simulink model "magnetometer"  (R2020b)
settings: Solver=VariableStepAuto  StartTime=0.0  StopTime=10.0  RelTol=1e-3
model mask{m_sf_cc=[1, 0, 0; 0, 1, 0; 0, 0, 1], m_bias=[0 0 0], m_noise=[0 0 0], m_sath=[inf inf inf], m_satl=[-inf -inf -inf], sample_rate=100}
  mask prompts: m_sf_cc "Scale factors and cross coupling:"; m_bias "Bias [uT]:"; m_noise "Noise [uT]:"; m_sath "Upper limits [uT]:"; m_satl "Lower limits [uT[:"; sample_rate "Sample rate [Hz]:"
model workspace (MAT data in the model file):
  m_bias = Simulink.Parameter
  m_bias.Value = [0 0 0]
  m_bias.DataType = 'auto'
  m_bias.Dimensions = [1 3]
  m_noise = Simulink.Parameter
  m_noise.Value = [0 0 0]
  m_noise.DataType = 'auto'
  m_noise.Dimensions = [1 3]
  m_sath = Simulink.Parameter
  m_sath.Value = [Inf Inf Inf]
  m_sath.DataType = 'auto'
  m_sath.Dimensions = [1 3]
  m_satl = Simulink.Parameter
  m_satl.Value = [-Inf -Inf -Inf]
  m_satl.DataType = 'auto'
  m_satl.Dimensions = [1 3]
  m_sf_cc = Simulink.Parameter
  m_sf_cc.Value = [1  0  0; 0  1  0; 0  0  1]
  m_sf_cc.DataType = 'auto'
  m_sf_cc.Dimensions = [3 3]
  sample_rate = Simulink.Parameter
  sample_rate.Value = 100
  sample_rate.DataType = 'auto'
  sample_rate.Dimensions = [1 1]
libraries: simulink x1
settings Model: ParameterArgumentNames=m_bias,m_noise,m_sath,m_satl,m_sf_cc,sample_rate  OrderedModelArguments=off  Creator=brian  LastModifiedBy=brian

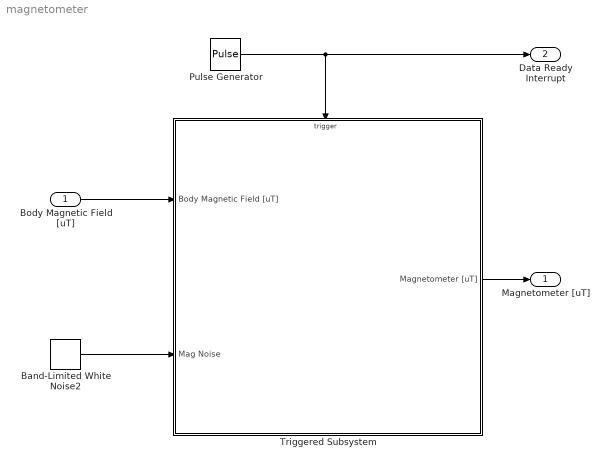
== system magnetometer ==
  Body Magnetic Field [uT] : Inport
  Band-Limited White Noise2 : simulink/Sources/Band-Limited White Noise  Cov=m_noise  Ts=0.1  seed=[23341]
  Pulse Generator : DiscretePulseGenerator  PulseType=Time based  Period=1/sample_rate  PulseWidth=5
  Triggered Subsystem : Subsystem  TreatAsAtomicUnit=on
  Magnetometer [uT] : Outport
  Data Ready Interrupt : Outport  Port=2
  wires:
  Band-Limited White Noise2/1 -> Triggered Subsystem/2(Mag Noise)
  Pulse Generator/1 -> Data Ready Interrupt/1, Triggered Subsystem/Trigger
  Triggered Subsystem/1(Magnetometer [uT]) -> Magnetometer [uT]/1
  Body Magnetic Field [uT]/1 -> Triggered Subsystem/1(Body Magnetic Field [uT])

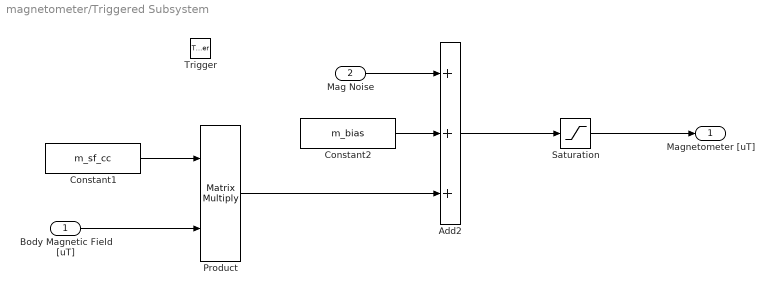
== system magnetometer/Triggered Subsystem ==
  Body Magnetic Field [uT] : Inport  PortDimensions=3
  Mag Noise : Inport  Port=2  PortDimensions=3
  Trigger : TriggerPort  VariantControl=Variant
  Add2 : Sum  Inputs=+++
  Constant1 : Constant  Value=m_sf_cc
  Constant2 : Constant  Value=m_bias
  Product : Product  Multiplication=Matrix(*)
  Saturation : Saturate  UpperLimit=m_sath  LowerLimit=m_satl
  Magnetometer [uT] : Outport  PortDimensions=3
  wires:
  Product/1 -> Add2/3
  Constant2/1 -> Add2/2
  Mag Noise/1 -> Add2/1
  Body Magnetic Field [uT]/1 -> Product/2
  Constant1/1 -> Product/1
  Add2/1 -> Saturation/1
  Saturation/1 -> Magnetometer [uT]/1
